simulink model "unit_and_Dunit_doubleRx"  (R2019b)
settings: Solver=VariableStepAuto  StartTime=0.0  StopTime=0.01  RelTol=1e-3
libraries: fl_lib x31, nesl_utility x24, ee_lib x12, powerlib_meascontrol x5, dspstat3 x3
settings Model: Creator=LRF  LastModifiedBy=LRF

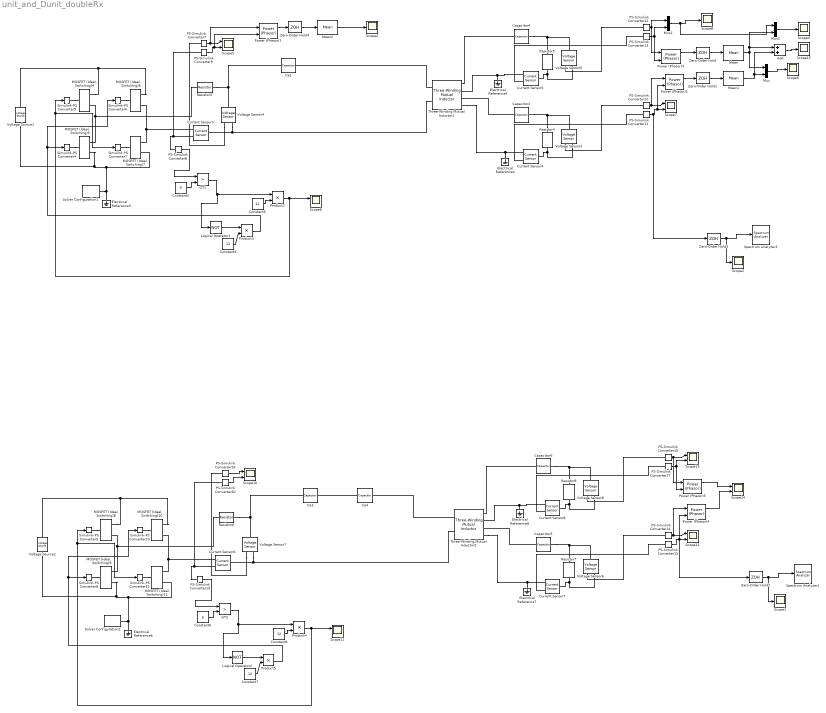
== system unit_and_Dunit_doubleRx ==
  Add : Sum
  Ca2 : fl_lib/Electrical/Electrical Elements/Capacitor  c=2.66 nF  r=1e-6 Ohm  g=0 1/Ohm  i_specify=off  i_priority=None  i=0 A  i_nominal_specify=off  i_nominal_unit=A  i_nominal_value=1  v_specify=off  v_priority=None  v=0 V  v_nominal_specify=off  v_nominal_unit=V  v_nominal_value=1  vc_specify=off  vc_priority=High  vc=0 V  vc_nominal_specify=off  vc_nominal_unit=V  vc_nominal_value=1
  Ca3 : fl_lib/Electrical/Electrical Elements/Capacitor  c=1517 pF  r=1e-6 Ohm  g=0 1/Ohm  i_specify=off  i_priority=None  i=0 A  i_nominal_specify=off  i_nominal_unit=A  i_nominal_value=1  v_specify=off  v_priority=None  v=0 V  v_nominal_specify=off  v_nominal_unit=V  v_nominal_value=1  vc_specify=off  vc_priority=High  vc=0 V  vc_nominal_specify=off  vc_nominal_unit=V  vc_nominal_value=1
  Ca4 : fl_lib/Electrical/Electrical Elements/Capacitor  c=1517 pF  r=1e-6 Ohm  g=0 1/Ohm  i_specify=off  i_priority=None  i=0 A  i_nominal_specify=off  i_nominal_unit=A  i_nominal_value=1  v_specify=off  v_priority=None  v=0 V  v_nominal_specify=off  v_nominal_unit=V  v_nominal_value=1  vc_specify=off  vc_priority=High  vc=0 V  vc_nominal_specify=off  vc_nominal_unit=V  vc_nominal_value=1
  Capacitor2 : fl_lib/Electrical/Electrical Elements/Capacitor  c=2.19 nF  r=1e-6 Ohm  g=0 1/Ohm  i_specify=off  i_priority=None  i=0 A  i_nominal_specify=off  i_nominal_unit=A  i_nominal_value=1  v_specify=off  v_priority=None  v=0 V  v_nominal_specify=off  v_nominal_unit=V  v_nominal_value=1  vc_specify=off  vc_priority=High  vc=0 V  vc_nominal_specify=off  vc_nominal_unit=V  vc_nominal_value=1
  Capacitor4 : fl_lib/Electrical/Electrical Elements/Capacitor  c=2.19 nF  r=1e-6 Ohm  g=0 1/Ohm  i_specify=off  i_priority=None  i=0 A  i_nominal_specify=off  i_nominal_unit=A  i_nominal_value=1  v_specify=off  v_priority=None  v=0 V  v_nominal_specify=off  v_nominal_unit=V  v_nominal_value=1  vc_specify=off  vc_priority=High  vc=0 V  vc_nominal_specify=off  vc_nominal_unit=V  vc_nominal_value=1
  Capacitor5 : fl_lib/Electrical/Electrical Elements/Capacitor  c=1013 pF  r=1e-6 Ohm  g=0 1/Ohm  i_specify=off  i_priority=None  i=0 A  i_nominal_specify=off  i_nominal_unit=A  i_nominal_value=1  v_specify=off  v_priority=None  v=0 V  v_nominal_specify=off  v_nominal_unit=V  v_nominal_value=1  vc_specify=off  vc_priority=High  vc=0 V  vc_nominal_specify=off  vc_nominal_unit=V  vc_nominal_value=1
  Capacitor6 : fl_lib/Electrical/Electrical Elements/Capacitor  c=1013 pF  r=1e-6 Ohm  g=0 1/Ohm  i_specify=off  i_priority=None  i=0 A  i_nominal_specify=off  i_nominal_unit=A  i_nominal_value=1  v_specify=off  v_priority=None  v=0 V  v_nominal_specify=off  v_nominal_unit=V  v_nominal_value=1  vc_specify=off  vc_priority=High  vc=0 V  vc_nominal_specify=off  vc_nominal_unit=V  vc_nominal_value=1
  Constant2 : Constant  Value=0
  Constant{4..5,7..8} (4 alike) : Constant  Value=12
  Constant6 : Constant  Value=0
  Current Sensor{3..8} (6 alike) : fl_lib/Electrical/Electrical Sensors/Current Sensor
  Electrical Reference{3..8} (6 alike) : fl_lib/Electrical/Electrical Elements/Electrical Reference
  GT1 : RelationalOperator  Operator=>  OutDataTypeStr=boolean  RndMeth=Simplest
  GT2 : RelationalOperator  Operator=>  OutDataTypeStr=boolean  RndMeth=Simplest
  Logical Operator1 : Logic  Operator=NOT  AllPortsSameDT=off  OutDataTypeStr=boolean
  Logical Operator2 : Logic  Operator=NOT  AllPortsSameDT=off  OutDataTypeStr=boolean
  MOSFET (Ideal, Switching){4..11} (8 alike) : ee_lib/Semiconductors & Converters/MOSFET (Ideal, Switching)  Rds=0.01 Ohm  Goff=1e-6 1/Ohm  Vth=2 V  diode_param=1  diode_Vf=0.8 V  diode_Ron=0.001 Ohm  diode_Goff=1e-5 1/Ohm  diode_C=50e-9 F  diode_iRM=-235 A  diode_iF=300 A  diode_idot=-50 A/us  diode_trr_param=1  diode_trr_factor=3  diode_trr=15 us  diode_Qrr=1500 s*uA  thermal_loss_option=2  Voff=300 V  Tau=1e-4 s  Tj=[298.15, 398.15] K  Iout_scalar=600 A  Eon_scalar=22.86e-3 J  Eoff_scalar=17.14e-3 J  Von_scalar=2.7 V  Iout_data=[0, 10, 50, 100, 200, 400, 600] A  Eon_data=[0, .29, 1.43, 2.86, 5.71, 13.14, 22.86; 0, .57, 2.63, 5.14, 10.29, 20.57, 30.29] * 1e-3 J  Eoff_data=[0, .21, 1.07, 2.14, 4.29, 9.86, 17.14; 0, .43, 1.97, 3.86, 7.71, 15.43, 22.71] * 1e-3 J  Von_data=[0, 1.1, 1.3, 1.45, 1.75, 2.25, 2.7; 0, 1, 1.15, 1.35, 1.7, 2.35, 3] V
      settings: SourceProductName=Simscape Electrical
  Mean : dspstat3/Mean  run=on  reset_popup=None  directionMode=Each column  dimension=1  roiEnable=off  roiType=Rectangles  roiPortion=Entire ROI  roiOutput=Individual statistics for each ROI  roiFlag=off  roundingMode=Floor  overflowMode=off  outputDataTypeStr=Inherit: Same as accumulator  outputMin=[]  outputMax=[]  outputLastDataTypeStr=Inherit: Same as accumulator
  Mean1 : dspstat3/Mean  run=on  reset_popup=None  directionMode=Each column  dimension=1  roiEnable=off  roiType=Rectangles  roiPortion=Entire ROI  roiOutput=Individual statistics for each ROI  roiFlag=off  roundingMode=Floor  overflowMode=off  outputDataTypeStr=Inherit: Same as accumulator  outputMin=[]  outputMax=[]  outputLastDataTypeStr=Inherit: Same as accumulator
  Mean2 : dspstat3/Mean  run=on  reset_popup=None  directionMode=Each column  dimension=1  roiEnable=off  roiType=Rectangles  roiPortion=Entire ROI  roiOutput=Individual statistics for each ROI  roiFlag=off  roundingMode=Floor  overflowMode=off  outputDataTypeStr=Inherit: Same as accumulator  outputMin=[]  outputMax=[]  outputLastDataTypeStr=Inherit: Same as accumulator
  Mux : Mux  Inputs=2
  Mux1 : Mux  Inputs=2
  Mux2 : Mux  Inputs=2
  PS-Simulink Converter{7..20} (14 alike) : nesl_utility/PS-Simulink Converter  PhysicalDomain=network_engine_domain  SubClassName=ps_output  LeftPortType=input  RightPortType=output  PseudoPeriodic=off  Frequencies=[]  Unit=inherit  AffineConversion=off
  Power (Phasor){1..5} (5 alike) : powerlib_meascontrol/Measurements/Power (Phasor)
      settings: SourceProductName=Simscape Electrical  SourceProductBaseCode=PS
  Product{2..5} (4 alike) : Product
  Resistor3 : fl_lib/Electrical/Electrical Elements/Resistor  R=0 Ohm  i_specify=off  i_priority=None  i=0 A  i_nominal_specify=off  i_nominal_unit=A  i_nominal_value=1  v_specify=off  v_priority=None  v=0 V  v_nominal_specify=off  v_nominal_unit=V  v_nominal_value=1
  Resistor4 : fl_lib/Electrical/Electrical Elements/Resistor  R=10 Ohm  i_specify=off  i_priority=None  i=0 A  i_nominal_specify=off  i_nominal_unit=A  i_nominal_value=1  v_specify=off  v_priority=None  v=0 V  v_nominal_specify=off  v_nominal_unit=V  v_nominal_value=1
  Resistor5 : fl_lib/Electrical/Electrical Elements/Resistor  R=10 Ohm  i_specify=off  i_priority=None  i=0 A  i_nominal_specify=off  i_nominal_unit=A  i_nominal_value=1  v_specify=off  v_priority=None  v=0 V  v_nominal_specify=off  v_nominal_unit=V  v_nominal_value=1
  Resistor6 : fl_lib/Electrical/Electrical Elements/Resistor  R=0 Ohm  i_specify=off  i_priority=None  i=0 A  i_nominal_specify=off  i_nominal_unit=A  i_nominal_value=1  v_specify=off  v_priority=None  v=0 V  v_nominal_specify=off  v_nominal_unit=V  v_nominal_value=1
  Resistor7 : fl_lib/Electrical/Electrical Elements/Resistor  R=15 Ohm  i_specify=off  i_priority=None  i=0 A  i_nominal_specify=off  i_nominal_unit=A  i_nominal_value=1  v_specify=off  v_priority=None  v=0 V  v_nominal_specify=off  v_nominal_unit=V  v_nominal_value=1
  Resistor8 : fl_lib/Electrical/Electrical Elements/Resistor  R=15 Ohm  i_specify=off  i_priority=None  i=0 A  i_nominal_specify=off  i_nominal_unit=A  i_nominal_value=1  v_specify=off  v_priority=None  v=0 V  v_nominal_specify=off  v_nominal_unit=V  v_nominal_value=1
  Scope{1..4,8..9,15} (7 alike) : Scope
  Scope{5..7,10..14} (8 alike) : Scope  NumInputPorts=2
  Simulink-PS Converter{4..11} (8 alike) : nesl_utility/Simulink-PS Converter  PhysicalDomain=network_engine_domain  SubClassName=ps_input  LeftPortType=input  RightPortType=output  PseudoPeriodic=off  Frequencies=[]  NoiseDistribution=none  NoiseParameters=[]  Unit=1  AffineConversion=off  FilteringAndDerivatives=provide  SimscapeFilterOrder=1  InputFilterTimeConstant=0.001  UdotUserProvided=0
  Solver Configuration1 : nesl_utility/Solver Configuration  PhysicalDomain=network_engine_domain  SubClassName=solver  LeftPortType=input  RightPortType=generic  Tones=[]  Harmonics=[]  SimulateNoise=off  Profile=off  UseLocalSampling=off  EnableSwitchedLinearOptims=on  FrequencyDomain=off  UseCCode=off  RelTol=0.001  AbsTol=1e-06  MinStep=1e-09  ToWorkspace=off  RevertToSquareIcSolve=off  NumHomotopyIterations=100  PhasorMode=off  PhasorModeNumHarmonics=1  DoDC=off  ResidualTolerance=1e-09  UseLocalSolver=off  LocalSolverChoice=NE_BACKWARD_EULER_ADVANCER  LocalSolverSampleTime=0.001  DoFixedCost=off  MaxNonlinIter=3  MaxModeIter=2  LinearAlgebra=auto  EquationFormulation=NE_TIME_EF  DelaysMemoryBudget=1024  AutomaticFiltering=on  FilteringTimeConstant=0.001  PartitionStorageMethod=AS_NEEDED  PartitionMemoryBudget=1024  PartitionMethod=ROBUST
  Solver Configuration2 : nesl_utility/Solver Configuration  PhysicalDomain=network_engine_domain  SubClassName=solver  LeftPortType=input  RightPortType=generic  Tones=[]  Harmonics=[]  SimulateNoise=off  Profile=off  UseLocalSampling=off  EnableSwitchedLinearOptims=on  FrequencyDomain=off  UseCCode=off  RelTol=0.001  AbsTol=1e-06  MinStep=1e-09  ToWorkspace=off  RevertToSquareIcSolve=off  NumHomotopyIterations=100  PhasorMode=off  PhasorModeNumHarmonics=1  DoDC=off  ResidualTolerance=1e-09  UseLocalSolver=off  LocalSolverChoice=NE_BACKWARD_EULER_ADVANCER  LocalSolverSampleTime=0.001  DoFixedCost=off  MaxNonlinIter=3  MaxModeIter=2  LinearAlgebra=auto  EquationFormulation=NE_TIME_EF  DelaysMemoryBudget=1024  AutomaticFiltering=on  FilteringTimeConstant=0.001  PartitionStorageMethod=AS_NEEDED  PartitionMemoryBudget=1024  PartitionMethod=ROBUST
  Spectrum Analyzer1 : SpectrumAnalyzer
  Spectrum Analyzer3 : SpectrumAnalyzer
  Three-Winding Mutual Inductor1 : ee_lib/Passive/Transformers/Three-Winding Mutual Inductor  L1=59.52 uH  L2=72.26 uH  L3=72.26 uH  K12=0.1  K13=0.1  K23=0  IC_given=1  IC1=0 A  IC2=0 A  IC3=0 A
      settings: SourceProductName=Simscape Electrical  SourceProductBaseCode=PS  InternalSimscapePortConfiguration="{\"Bottom\":[],\"Left\":[{\"id\":\"p1\",\"label\":\"1+\",\"type\":\"foundation.electrical.electrical\"},{\"id\":\"n1\",\"label\":\"1-\",\"type\":\"foundation.electrical.electrical\"}],\"Right\":[{\"id\":\"p2\",\"label\":\"2+\",\"type\":\"foundation.electrical.electrical\"},{\"id\":\"n2\",\"label\":\"2-\",\"type\":\"foundation.electrical.electrical\"},{\"id\":\"p3\",\"label\":\"3+\",\"type\":\"foundation.electrical.electrical\"},{\"id\":\"n3\",\"label\":\"3-\",\"type\":\"foundation.electrical.electrical\"}],\"Top\":[]}"
  Three-Winding Mutual Inductor2 : ee_lib/Passive/Transformers/Three-Winding Mutual Inductor  L1=133.58 uH  L2=100 uH  L3=100 uH  K12=0.1  K13=0.1  K23=0  IC_given=1  IC1=0 A  IC2=0 A  IC3=0 A
      settings: SourceProductName=Simscape Electrical  SourceProductBaseCode=PS  InternalSimscapePortConfiguration="{\"Bottom\":[],\"Left\":[{\"id\":\"p1\",\"label\":\"1+\",\"type\":\"foundation.electrical.electrical\"},{\"id\":\"n1\",\"label\":\"1-\",\"type\":\"foundation.electrical.electrical\"}],\"Right\":[{\"id\":\"p2\",\"label\":\"2+\",\"type\":\"foundation.electrical.electrical\"},{\"id\":\"n2\",\"label\":\"2-\",\"type\":\"foundation.electrical.electrical\"},{\"id\":\"p3\",\"label\":\"3+\",\"type\":\"foundation.electrical.electrical\"},{\"id\":\"n3\",\"label\":\"3-\",\"type\":\"foundation.electrical.electrical\"}],\"Top\":[]}"
  Voltage Sensor{3..8} (6 alike) : fl_lib/Electrical/Electrical Sensors/Voltage Sensor
  Voltage Source1 : ee_lib/Sources/Voltage Source  dc_voltage=48 V  ac_voltage=0 V  ac_shift=0 rad  ac_frequency=60 Hz  noise_mode=0  PSD=0 V^2/Hz  repeatability=1  auto_seed=508128604  user_seed=0  sample_time=1e-3 s  i_specify=off  i_priority=None  i=0 A  i_nominal_specify=off  i_nominal_unit=A  i_nominal_value=1  v_specify=off  v_priority=None  v=0 V  v_nominal_specify=off  v_nominal_unit=V  v_nominal_value=1
      settings: SourceProductName=Simscape Electrical
  Voltage Source2 : ee_lib/Sources/Voltage Source  dc_voltage=15 V  ac_voltage=0 V  ac_shift=0 rad  ac_frequency=60 Hz  noise_mode=0  PSD=0 V^2/Hz  repeatability=1  auto_seed=746822400  user_seed=0  sample_time=1e-3 s  i_specify=off  i_priority=None  i=0 A  i_nominal_specify=off  i_nominal_unit=A  i_nominal_value=1  v_specify=off  v_priority=None  v=0 V  v_nominal_specify=off  v_nominal_unit=V  v_nominal_value=1
      settings: SourceProductName=Simscape Electrical
  Zero-Order Hold : ZeroOrderHold  SampleTime=-1
  Zero-Order Hold1 : ZeroOrderHold  SampleTime=-1
  Zero-Order Hold2 : ZeroOrderHold  SampleTime=1e-7
  Zero-Order Hold3 : ZeroOrderHold  SampleTime=1e-7
  Zero-Order Hold4 : ZeroOrderHold  SampleTime=-1
  wires:
  PS-Simulink Converter7/1 -> Power (Phasor)1/1, Scope5/1
  PS-Simulink Converter9/1 -> Power (Phasor)1/2, Scope5/2
  PS-Simulink Converter8/1 -> GT1/1
  PS-Simulink Converter13/1 -> Power (Phasor)3/2, Mux1/2
  GT1/1 -> Logical Operator1/1, Product2/1
  PS-Simulink Converter10/1 -> Power (Phasor)2/1, Scope7/1
  Product2/1 -> Simulink-PS Converter7/1, Simulink-PS Converter5/1, Scope6/1
  Logical Operator1/1 -> Product3/1
  Product3/1 -> Simulink-PS Converter6/1, Simulink-PS Converter4/1
  Constant2/1 -> GT1/2
  Constant5/1 -> Product2/2
  Constant4/1 -> Product3/2
  PS-Simulink Converter12/1 -> Power (Phasor)3/1, Mux1/1
  Product5/1 -> Simulink-PS Converter10/1, Simulink-PS Converter8/1
  Logical Operator2/1 -> Product5/1
  GT2/1 -> Logical Operator2/1, Product4/1
  PS-Simulink Converter18/1 -> Scope10/1
  PS-Simulink Converter17/1 -> Power (Phasor)5/2, Scope13/2
  PS-Simulink Converter20/1 -> Scope10/2
  PS-Simulink Converter19/1 -> GT2/1
  Constant8/1 -> Product4/2
  Product4/1 -> Simulink-PS Converter11/1, Simulink-PS Converter9/1, Scope11/1
  PS-Simulink Converter16/1 -> Power (Phasor)5/1, Scope13/1
  PS-Simulink Converter14/1 -> Power (Phasor)4/1, Scope12/1
  Constant6/1 -> GT2/2
  Constant7/1 -> Product5/2
  Power (Phasor)5/1 -> Scope14/1
  Power (Phasor)4/1 -> Scope14/2
  PS-Simulink Converter15/1 -> Zero-Order Hold2/1, Power (Phasor)4/2, Scope12/2
  Zero-Order Hold2/1 -> Scope1/1, Spectrum Analyzer1/1
  PS-Simulink Converter11/1 -> Zero-Order Hold3/1, Power (Phasor)2/2, Scope7/2
  Zero-Order Hold3/1 -> Scope2/1, Spectrum Analyzer3/1
  Zero-Order Hold/1 -> Mean/1
  Power (Phasor)3/1 -> Zero-Order Hold/1
  Power (Phasor)2/1 -> Zero-Order Hold1/1
  Zero-Order Hold1/1 -> Mean1/1
  Mean/1 -> Add/1, Mux2/2, Mux/1
  Mean1/1 -> Add/2, Mux/2
  Mux/1 -> Scope9/1
  Mux1/1 -> Mux2/1, Scope8/1
  Mux2/1 -> Scope3/1
  Zero-Order Hold4/1 -> Mean2/1
  Power (Phasor)1/1 -> Zero-Order Hold4/1
  Mean2/1 -> Scope4/1
  Add/1 -> Scope15/1
  connections:
  Current Sensor4/RConn2 -- Electrical Reference4/LConn1 -- Three-Winding Mutual Inductor1/RConn4
  Three-Winding Mutual Inductor1/RConn2 -- Current Sensor5/RConn2 -- Electrical Reference5/LConn1
  Resistor4/LConn1 -- Capacitor2/RConn1 -- Voltage Sensor3/LConn1
  Voltage Sensor4/LConn1 -- Resistor3/RConn1 -- Ca2/LConn1
  Current Sensor5/LConn1 -- Resistor5/RConn1 -- Voltage Sensor5/RConn2
  "MOSFET (Ideal, Switching)6"/RConn1 -- "MOSFET (Ideal, Switching)4"/RConn1 -- Voltage Source1/LConn1
  "MOSFET (Ideal, Switching)6"/RConn2 -- "MOSFET (Ideal, Switching)7"/RConn1 -- Current Sensor3/RConn2
  Three-Winding Mutual Inductor1/LConn1 -- Ca2/RConn1
  Resistor3/LConn1 -- "MOSFET (Ideal, Switching)5"/RConn1 -- "MOSFET (Ideal, Switching)4"/RConn2
  PS-Simulink Converter8/LConn1 -- Current Sensor3/RConn1 -- PS-Simulink Converter9/LConn1
  Voltage Sensor5/LConn1 -- Resistor5/LConn1 -- Capacitor4/RConn1
  Current Sensor3/LConn1 -- Voltage Sensor4/RConn2 -- Three-Winding Mutual Inductor1/LConn2
  "MOSFET (Ideal, Switching)7"/RConn2 -- Solver Configuration1/RConn1 -- Electrical Reference3/LConn1 -- "MOSFET (Ideal, Switching)5"/RConn2 -- Voltage Source1/RConn1
  Resistor4/RConn1 -- Voltage Sensor3/RConn2 -- Current Sensor4/LConn1
  Capacitor4/LConn1 -- Three-Winding Mutual Inductor1/RConn1
  PS-Simulink Converter12/LConn1 -- Voltage Sensor5/RConn1
  Simulink-PS Converter5/RConn1 -- "MOSFET (Ideal, Switching)4"/LConn1
  Simulink-PS Converter4/RConn1 -- "MOSFET (Ideal, Switching)5"/LConn1
  Current Sensor4/RConn1 -- PS-Simulink Converter11/LConn1
  Simulink-PS Converter7/RConn1 -- "MOSFET (Ideal, Switching)7"/LConn1
  Simulink-PS Converter6/RConn1 -- "MOSFET (Ideal, Switching)6"/LConn1
  Current Sensor5/RConn1 -- PS-Simulink Converter13/LConn1
  Voltage Sensor4/RConn1 -- PS-Simulink Converter7/LConn1
  Capacitor2/LConn1 -- Three-Winding Mutual Inductor1/RConn3
  PS-Simulink Converter10/LConn1 -- Voltage Sensor3/RConn1
  Resistor7/RConn1 -- Voltage Sensor6/RConn2 -- Current Sensor7/LConn1
  "MOSFET (Ideal, Switching)10"/RConn1 -- "MOSFET (Ideal, Switching)8"/RConn1 -- Voltage Source2/LConn1
  Current Sensor6/LConn1 -- Voltage Sensor7/RConn2 -- Three-Winding Mutual Inductor2/LConn2
  Voltage Sensor7/LConn1 -- Resistor6/RConn1 -- Ca3/LConn1
  Resistor7/LConn1 -- Capacitor5/RConn1 -- Voltage Sensor6/LConn1
  Voltage Source2/RConn1 -- "MOSFET (Ideal, Switching)9"/RConn2 -- Solver Configuration2/RConn1 -- Electrical Reference6/LConn1 -- "MOSFET (Ideal, Switching)11"/RConn2
  Current Sensor7/RConn2 -- Electrical Reference7/LConn1 -- Three-Winding Mutual Inductor2/RConn4
  Resistor6/LConn1 -- "MOSFET (Ideal, Switching)9"/RConn1 -- "MOSFET (Ideal, Switching)8"/RConn2
  Three-Winding Mutual Inductor2/RConn2 -- Current Sensor8/RConn2 -- Electrical Reference8/LConn1
  Current Sensor8/LConn1 -- Resistor8/RConn1 -- Voltage Sensor8/RConn2
  PS-Simulink Converter19/LConn1 -- Current Sensor6/RConn1 -- PS-Simulink Converter20/LConn1
  Voltage Sensor8/LConn1 -- Resistor8/LConn1 -- Capacitor6/RConn1
  "MOSFET (Ideal, Switching)10"/RConn2 -- "MOSFET (Ideal, Switching)11"/RConn1 -- Current Sensor6/RConn2
  Simulink-PS Converter10/RConn1 -- "MOSFET (Ideal, Switching)10"/LConn1
  Voltage Sensor7/RConn1 -- PS-Simulink Converter18/LConn1
  Capacitor5/LConn1 -- Three-Winding Mutual Inductor2/RConn3
  Simulink-PS Converter11/RConn1 -- "MOSFET (Ideal, Switching)11"/LConn1
  Current Sensor8/RConn1 -- PS-Simulink Converter17/LConn1
  PS-Simulink Converter16/LConn1 -- Voltage Sensor8/RConn1
  Capacitor6/LConn1 -- Three-Winding Mutual Inductor2/RConn1
  Current Sensor7/RConn1 -- PS-Simulink Converter15/LConn1
  PS-Simulink Converter14/LConn1 -- Voltage Sensor6/RConn1
  Simulink-PS Converter9/RConn1 -- "MOSFET (Ideal, Switching)8"/LConn1
  Simulink-PS Converter8/RConn1 -- "MOSFET (Ideal, Switching)9"/LConn1
  Three-Winding Mutual Inductor2/LConn1 -- Ca4/RConn1
  Ca4/LConn1 -- Ca3/RConn1
